simulink model "modele_lineaire_dec"  (R2021a)
settings: Solver=VariableStepAuto  StartTime=0.0  StopTime=tfin  RelTol=1e-10
values from neighbouring files (symbols this model uses):
  A_phi = [A_plaque(1,1),    A_plaque(1,4),  A_plaque(1,7) ... (first row only)    [decouplage.m]
  A_teta = [A_plaque(2,2),    A_plaque(2,5),  A_plaque(2,8) ... (first row only)    [decouplage.m]
  A_x = [A_sphere(1,1), A_sphere(1,3) ... (first row only)    [decouplage.m]
  A_y = [A_sphere(2,2), A_sphere(2,4) ... (first row only)    [decouplage.m]
  A_z = [A_plaque(3,3),    A_plaque(3,6),  A_plaque(3,9) ... (first row only)    [decouplage.m]
  B_phi = [            0 ... (first row only)    [decouplage.m]
  B_teta = [             0 ... (first row only)    [decouplage.m]
  B_x = [            0 ... (first row only)    [decouplage.m]
  B_y = [             0 ... (first row only)    [decouplage.m]
  B_z = [             0 ... (first row only)    [decouplage.m]
  C_phi = [C_plaque(1,1), 0,  0]    [decouplage.m]
  C_teta = [C_plaque(1,1), 0,  0]    [decouplage.m]
  C_x = [C_sphere(1,1), C_sphere(1,3) ... (first row only)    [decouplage.m]
  C_y = [C_sphere(2,2), C_sphere(2,4) ... (first row only)    [decouplage.m]
  C_z = [C_plaque(1,1), 0,  0]    [decouplage.m]
  D_phi = [0]    [decouplage.m]
  D_teta = [0]    [decouplage.m]
  D_x = [ 0;  0]    [decouplage.m]
  D_y = [ 0;  0]    [decouplage.m]
  D_z = [0]    [decouplage.m]
  V_eq = -4.9999    [decouplage.m]
settings Model: Creator=User  LastModifiedBy=Utilisateur
settings SolverCC: AlgebraicLoopSolver=LineSearch
settings DebuggingCC: SignalInfNanChecking=error

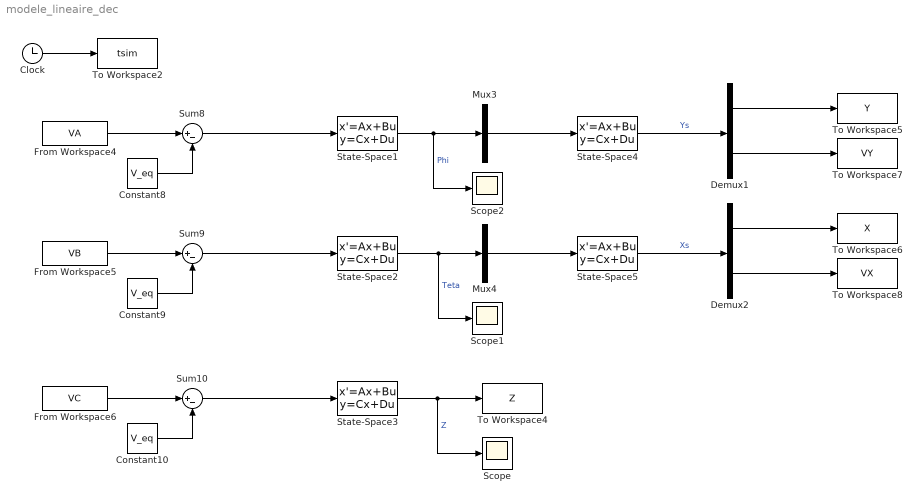
== system modele_lineaire_dec ==
  Clock : Clock
  Constant10 : Constant  Value=V_eq
  Constant8 : Constant  Value=V_eq
  Constant9 : Constant  Value=V_eq
  Demux1 : Demux  Outputs=2
  Demux2 : Demux  Outputs=2
  From Workspace4 : FromWorkspace  VariableName=VA
  From Workspace5 : FromWorkspace  VariableName=VB
  From Workspace6 : FromWorkspace  VariableName=VC
  Mux3 : Mux  Inputs=1
  Mux4 : Mux  Inputs=1
  Scope : Scope
  Scope1 : Scope
  Scope2 : Scope
  State-Space1 : StateSpace  A=A_phi  B=B_phi  C=C_phi  D=D_phi  InitialCondition=0  AbsoluteTolerance=1e-10
  State-Space2 : StateSpace  A=A_teta  B=B_teta  C=C_teta  D=D_teta  InitialCondition=0  AbsoluteTolerance=1e-10
  State-Space3 : StateSpace  A=A_z  B=B_z  C=C_z  D=D_z  InitialCondition=0  AbsoluteTolerance=1e-10
  State-Space4 : StateSpace  A=A_y  B=B_y  C=C_y  D=D_y  InitialCondition=0  AbsoluteTolerance=1e-10
  State-Space5 : StateSpace  A=A_x  B=B_x  C=C_x  D=D_x  InitialCondition=0  AbsoluteTolerance=1e-10
  Sum10 : Sum  Inputs=|+-
  Sum8 : Sum  Inputs=|+-
  Sum9 : Sum  Inputs=|+-
  To Workspace2 : ToWorkspace  VariableName=tsim  SampleTime=-1
  To Workspace4 : ToWorkspace  VariableName=Z  SampleTime=-1
  To Workspace5 : ToWorkspace  VariableName=Y  SampleTime=-1
  To Workspace6 : ToWorkspace  VariableName=X  SampleTime=-1
  To Workspace7 : ToWorkspace  VariableName=VY  SampleTime=-1
  To Workspace8 : ToWorkspace  VariableName=VX  SampleTime=-1
  wires:
  Clock/1 -> To Workspace2/1
  Constant10/1 -> Sum10/2
  From Workspace5/1 -> Sum9/1
  Constant8/1 -> Sum8/2
  From Workspace6/1 -> Sum10/1
  From Workspace4/1 -> Sum8/1
  Constant9/1 -> Sum9/2
  Sum8/1 -> State-Space1/1
  Sum9/1 -> State-Space2/1
  Sum10/1 -> State-Space3/1
  State-Space3/1 -> Scope/1, To Workspace4/1  "Z"
  Mux3/1 -> State-Space4/1
  State-Space1/1 -> Scope2/1, Mux3/1  "Phi"
  Mux4/1 -> State-Space5/1
  State-Space2/1 -> Scope1/1, Mux4/1  "Teta"
  State-Space4/1 -> Demux1/1  "Ys"
  Demux1/1 -> To Workspace5/1
  Demux1/2 -> To Workspace7/1
  State-Space5/1 -> Demux2/1  "Xs"
  Demux2/2 -> To Workspace8/1
  Demux2/1 -> To Workspace6/1
